simulink model "plant_open_loop_test"  (R2026a)
settings: Solver=VariableStepAuto  StopTime=300
model workspace (MAT data in the model file):
  test_front_drive_torque_Nm = 1
undefined symbols (not defined in the file): test_braking_cmd, test_drive_torque_Nm, test_road_friction_mu, test_slope, test_steering_wheel_deg
settings Model: Creator=rayyu  LastModifiedBy=rayyu

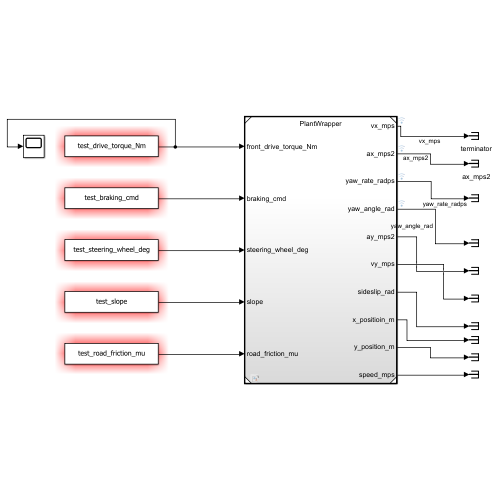
[thumbnail: Simulink's stored preview of the top-level diagram]
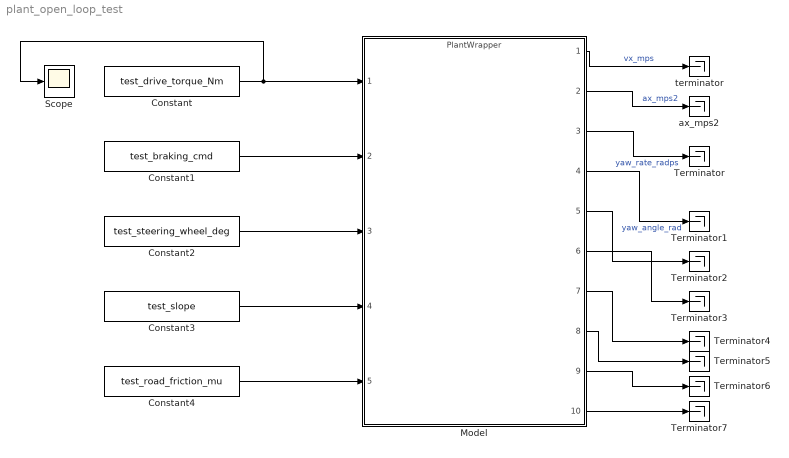
== system plant_open_loop_test ==
  Constant : Constant  Value=test_drive_torque_Nm  VectorParams1D=off  SampleTime=0.01
  Constant1 : Constant  Value=test_braking_cmd
  Constant2 : Constant  Value=test_steering_wheel_deg
  Constant3 : Constant  Value=test_slope
  Constant4 : Constant  Value=test_road_friction_mu
  Model : ModelReference  ModelNameDialog=PlantWrapper.slx  SimulationMode=Normal  ModelReferenceVersion=1.10
  Scope : Scope
      settings: ActiveDisplayYMinimum=9  ActiveDisplayYMaximum=11
  Terminator{,1..7} (8 alike) : Terminator
  ax_mps2 : Terminator
  terminator : Terminator
  wires:
  Constant/1 -> Scope/1, Model/1
  Constant1/1 -> Model/2
  Constant2/1 -> Model/3
  Constant3/1 -> Model/4
  Constant4/1 -> Model/5
  Model/1 -> terminator/1  "vx_mps"
  Model/2 -> ax_mps2/1  "ax_mps2"
  Model/3 -> Terminator/1  "yaw_rate_radps"
  Model/4 -> Terminator1/1  "yaw_angle_rad"
  Model/5 -> Terminator2/1
  Model/6 -> Terminator3/1
  Model/7 -> Terminator4/1
  Model/8 -> Terminator5/1
  Model/9 -> Terminator6/1
  Model/10 -> Terminator7/1
